simulink subsystem "AutomatedManualTransmission"  (R2023a)
settings: Solver=VariableStepAuto  StartTime=0.0  StopTime=10.0  RelTol=1e-3
undefined symbols (not defined in the file): PlntDriveshftDamp, PlntDriveshftStiff, PlntTransCltchRadius, PlntTransEffTempBpt, PlntTransGearRatioVect
libraries: autolibtransamt x1, autolibsharedcoupling x1
settings Model: Creator=The MathWorks, Inc.  LastModifiedBy=The MathWorks, Inc.
settings SolverCC: MaxZcPerStep=1
settings ModelReferenceCC: EnableRefExpFcnMdlSchedulingChecks=on

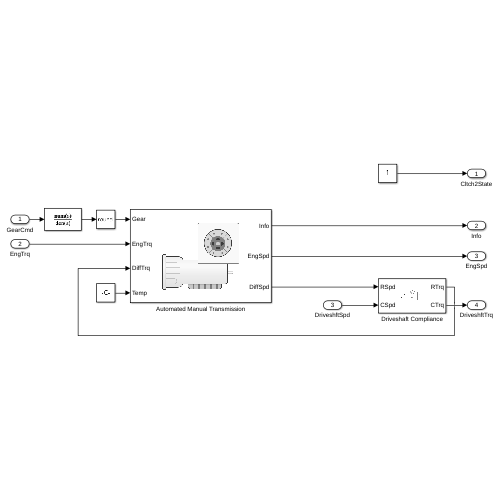
[thumbnail: Simulink's stored preview of the top-level diagram]
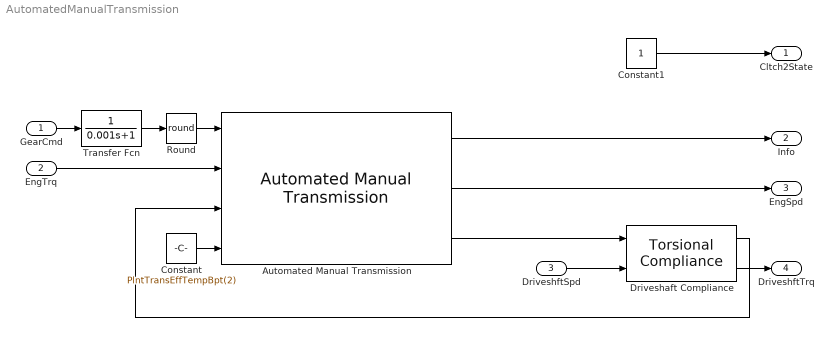
== system AutomatedManualTransmission ==
  GearCmd : Inport
  EngTrq : Inport  Port=2
  DriveshftSpd : Inport  Port=3
  Automated Manual Transmission : autolibtransamt/Automated Manual Transmission  VariantControl=1  cntrlType=Ideal integrated controller  TransEffModelPopup=Gear, input torque, input speed, and temperature  Jin=PlntTransInInertia  bin=PlntTransInDamp  omegain_o=PlntTransInitInVel  G=PlntTransGearNumVect  Trq_bpts=PlntTransEffTrqBpt  omega_bpts=PlntTransEffSpdBpt  Temp_bpts=PlntTransEffTempBpt  N=PlntTransGearRatioVect  Jout=PlntTransInertiaVect  bout=PlntTransDampVect  eta=PlntTransEffVect  eta_tbl=PlntTransEffTbl  omegaout_o=PlntTransInitOutVel  G_o=PlntTransInitGear  tauc=PlntTransCltchPrsTimeCnst  ts=PlntTransCltchSyncTime  tc=PlntTransCltchTime  R=PlntTransCltchRadius  K_c=PlntTransCltchForceGain  mus=PlntTransCltchStatFric  muk=PlntTransCltchKinFric  ClutchLocked=off  SynchLocked=off  maxAbsSpd=5e3
  Constant : Constant  Value=PlntTransEffTempBpt(2)  SampleTime=-1
  Constant1 : Constant  SampleTime=-1
  Driveshaft Compliance : autolibsharedcoupling/Torsional Compliance  port_config=Simulink  extInfo=off  k=PlntDriveshftStiff  b=PlntDriveshftDamp  theta_o=PlntDriveshftInitDeflect  domega_o=PlntDriveshftInitVel  omega_c=PlntDriveshftDampCutoffFreq  blkID=0  aMode=1
      settings: SourceProductName=Powertrain Blockset
  Round : Rounding  Operator=round
  Transfer Fcn : TransferFcn  Denominator=[0.001 1]
  Cltch2State : Outport  VectorParamsAs1DForOutWhenUnconnected=off
  Info : Outport  Port=2  VectorParamsAs1DForOutWhenUnconnected=off
  EngSpd : Outport  Port=3  VectorParamsAs1DForOutWhenUnconnected=off
  DriveshftTrq : Outport  Port=4  VectorParamsAs1DForOutWhenUnconnected=off
  wires:
  DriveshftSpd/1 -> Driveshaft Compliance/2
  EngTrq/1 -> Automated Manual Transmission/2
  Automated Manual Transmission/1 -> Info/1
  Driveshaft Compliance/1 -> Automated Manual Transmission/3
  Automated Manual Transmission/3 -> Driveshaft Compliance/1
  Constant1/1 -> Cltch2State/1
  Driveshaft Compliance/2 -> DriveshftTrq/1
  Automated Manual Transmission/2 -> EngSpd/1
  GearCmd/1 -> Transfer Fcn/1
  Constant/1 -> Automated Manual Transmission/4
  Round/1 -> Automated Manual Transmission/1
  Transfer Fcn/1 -> Round/1
